simulink model "LEGO_NXT_M1V4_Open_Loop_DC_Motor_Position"  (R2017a)
settings: Solver=FixedStepDiscrete  StartTime=0.0  StopTime=45  FixedStep=.003  RelTol=1e-3  EnableMultiTasking=on
libraries: MinSegLibrary_M1V4 x2
settings Model: SimulationMode=external  ExtModeTrigDuration=2  Creator=malcoj2  LastModifiedBy=mkupilik
settings DataIOCC: LimitDataPoints=on  SaveFormat=Array
settings OptimizationCC: PassReuseOutputArgsThreshold=0  MaxStackSize=64
settings DebuggingCC: UnderspecifiedInitializationDetection=Classic  MergeDetectMultiDrivingBlocksExec=none  ParameterTunabilityLossMsg=error  StateNameClashWarn=warning  SFUnexpectedBacktrackingDiag=warning  SFNoUnconditionalDefaultTransitionDiag=warning  SFExecutionAtInitializationDiag=none
settings HardwareCC: ProdBitPerInt=16  ProdBitPerPointer=16  ProdBitPerSizeT=16  ProdBitPerPtrDiffT=16  ProdLargestAtomicFloat=None  ProdWordSize=8  ProdHWDeviceType=Atmel->AVR  UseEmbeddedCoderFeatures=off
settings ModelReferenceCC: PropagateSignalLabelsOutOfModel=off
settings SFSimCC: MATLABDynamicMemAlloc=off
settings RTWCC: SystemTargetFile=ert.tlc  HardwareBoard=Arduino Mega 2560  TLCOptions=-aInlineSetEventsForThisBaseRateFcn=TLC_FALSE -aSuppressMultiTaskScheduler=TLC_FALSE -aRateBasedStepFcn=1  TemplateMakefile=ert_default_tmf  Description=Embedded Coder  GenerateReport=on  RTWVerbose=off  Toolchain=Arduino AVR  BuildConfiguration=Faster Runs  LaunchReport=on
settings CodeAppCC: ForceParamTrailComments=on  OperatorAnnotations=on  MATLABSourceComments=on
settings ERTTargetCC: ERTCustomFileBanners=off  SupportContinuousTime=on  SupportNonInlinedSFcns=on  RemoveResetFunc=off  SupportVariableSizeSignals=on  ModelStepFunctionPrototypeControlCompliant=off
settings ConfigComp: CovMetricSettings=dw  CovHtmlReporting=on  CovSaveCumulativeToWorkspaceVar=on  CovSaveSingleToWorkspaceVar=on  CovExternalEMLEnable=off

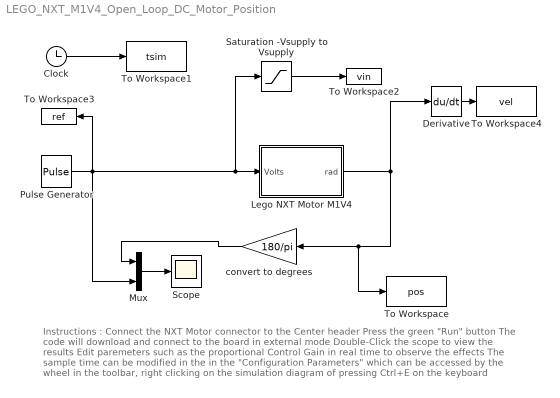
== system LEGO_NXT_M1V4_Open_Loop_DC_Motor_Position ==
  note: Instructions :
      | Connect the NXT Motor connector to the Center header
      | Press the green "Run" button
      | The code will download and connect to the board in external mode
      | Double-Click the scope to view the results
      | Edit paremeters such as the proportional Control Gain in real time to observe the effects
      |
      | The sample time can be modified in the in the "Configuration Parameters" which can be accessed by the wheel in the toolbar, right clicking on the simulation diagram of pressing Ctrl+E on the keyboard
  Clock : Clock
  Derivative : Derivative
  Lego NXT Motor M1V4 : Subsystem
  Mux : Mux  Inputs=2
  Pulse Generator : DiscretePulseGenerator  PulseType=Time based  Amplitude=90  Period=3  PulseWidth=50
  Saturation -Vsupply to Vsupply : Saturate  UpperLimit=3.25  LowerLimit=-3.25  OutDataTypeStr=single
  Scope : Scope
  To Workspace : ToWorkspace  VariableName=pos  SampleTime=-1
  To Workspace1 : ToWorkspace  VariableName=tsim  SampleTime=-1
  To Workspace2 : ToWorkspace  VariableName=vin  SampleTime=-1
  To Workspace3 : ToWorkspace  VariableName=ref  SampleTime=-1
  To Workspace4 : ToWorkspace  VariableName=vel  SampleTime=-1
  convert to degrees : Gain  Gain=180/pi
  wires:
  Clock/1 -> To Workspace1/1
  convert to degrees/1 -> Mux/1
  Mux/1 -> Scope/1
  Pulse Generator/1 -> Saturation -Vsupply to Vsupply/1, Lego NXT Motor M1V4/1(Volts), Mux/2, To Workspace3/1
  Saturation -Vsupply to Vsupply/1 -> To Workspace2/1
  Derivative/1 -> To Workspace4/1
  Lego NXT Motor M1V4/1(rad) -> Derivative/1, To Workspace/1, convert to degrees/1

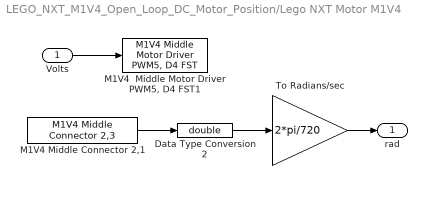
== system LEGO_NXT_M1V4_Open_Loop_DC_Motor_Position/Lego NXT Motor M1V4 ==
  Volts : Inport
  Data Type Conversion2 : DataTypeConversion  OutDataTypeStr=double
  "M1V4  Middle Motor Driver PWM5, D4 FST1" : MinSegLibrary_M1V4/M1V4  Middle Motor Driver PWM5, D4 FST  Vsupply=3.25
  M1V4 Middle Connector 2,1 : MinSegLibrary_M1V4/M1V4 Middle Connector 2,3  Encoder=0  PinA=3  PinB=2  PWMFSelect=3  PWMTimer=-1
  To Radians/sec : Gain  Gain=2*pi/720
  rad : Outport
  wires:
  To Radians/sec/1 -> rad/1
  M1V4 Middle Connector 2,1/1 -> Data Type Conversion2/1
  Volts/1 -> "M1V4  Middle Motor Driver PWM5, D4 FST1"/1
  Data Type Conversion2/1 -> To Radians/sec/1
